simulink model "Desacople_RetroA_Lazo_Incorporacion_Torque"  (R2023b)
settings: Solver=VariableStepAuto  StartTime=0.0  StopTime=10.0  RelTol=1e-3
values from neighbouring files (symbols this model uses):
  lambda_m = 0.016    [parametros_proyecto2.m]
  Ld = 6.6e-3    (= 0.0066)    [parametros_proyecto2.m]
  Lq = 5.8e-3    (= 0.0058)    [parametros_proyecto2.m]
  r = 120    [parametros_proyecto2.m]
undefined symbols (not defined in the file or in its folder): b_eq, k_l, P_p
settings Model: Creator=ignab  LastModifiedBy=ignab

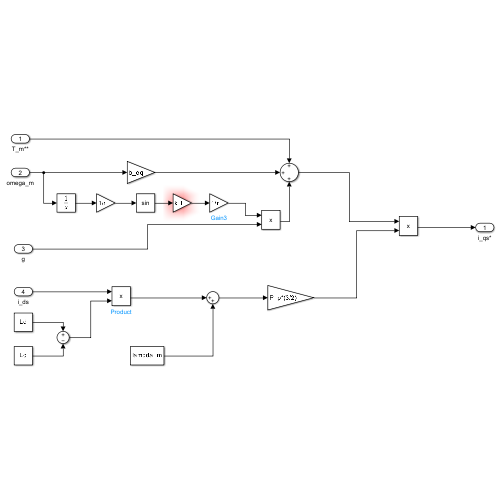
[thumbnail: Simulink's stored preview of the top-level diagram]
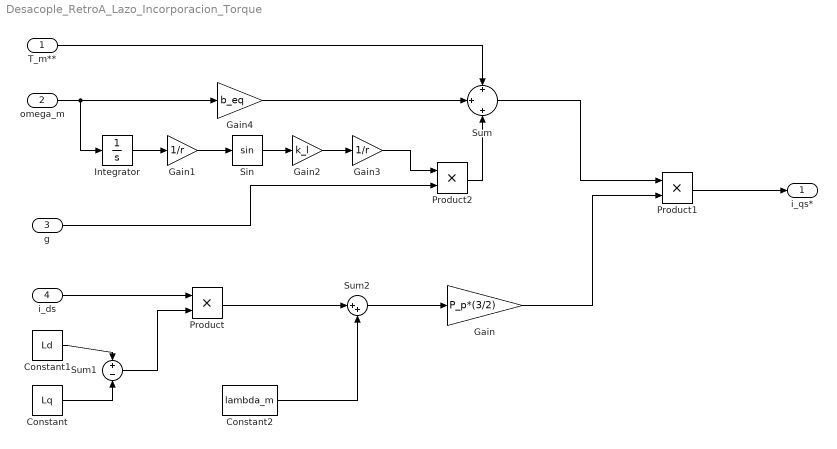
== system Desacople_RetroA_Lazo_Incorporacion_Torque ==
  T_m** : Inport
  omega_m : Inport  Port=2
  g : Inport  Port=3
  i_ds : Inport  Port=4
  Constant : Constant  Value=Lq
  Constant1 : Constant  Value=Ld
  Constant2 : Constant  Value=lambda_m
  Gain : Gain  Gain=P_p*(3/2)
  Gain1 : Gain  Gain=1/r
  Gain2 : Gain  Gain=k_l
  Gain3 : Gain  Gain=1/r
  Gain4 : Gain  Gain=b_eq
  Integrator : Integrator
  Product : Product
  Product1 : Product
  Product2 : Product
  Sin : Trigonometry
  Sum : Sum  Inputs=+|+|+
  Sum1 : Sum  Inputs=+|-
  Sum2 : Sum  Inputs=|++
  i_qs* : Outport
  wires:
  Constant/1 -> Sum1/2
  Constant1/1 -> Sum1/1
  Sum1/1 -> Product/2
  Product/1 -> Sum2/1
  i_ds/1 -> Product/1
  Constant2/1 -> Sum2/2
  Sum2/1 -> Gain/1
  Gain/1 -> Product1/2
  Product1/1 -> i_qs*/1
  Sum/1 -> Product1/1
  Product2/1 -> Sum/3
  g/1 -> Product2/2
  Gain2/1 -> Gain3/1
  Sin/1 -> Gain2/1
  Gain1/1 -> Sin/1
  Integrator/1 -> Gain1/1
  Gain3/1 -> Product2/1
  omega_m/1 -> Integrator/1, Gain4/1
  Gain4/1 -> Sum/2
  T_m**/1 -> Sum/1
